simulink model "fusionAlg"  (R2018b)
settings: Solver=FixedStepDiscrete  StartTime=0.0  StopTime=inf  FixedStep=0.01  RelTol=1e-3
PostLoadFcn:
  | if any(exist('dsrtsu_mdlpostloadfcn', 'file') ~= 0), dsrtsu_mdlpostloadfcn('Execute', bdroot); end
model workspace (MAT data in the model file):
  handle : class17 (value not decoded)
(part 5 of 24)

== system fusionAlg/FUSION /FUS_DataAdapter/VisionAdapter/LaneAdapter/Lane_ProtA ==
  EyeQ4_ProtA : Inport
  Bus Creator1 : BusCreator  Inputs=15  OutDataTypeStr=Bus: FUS_EYEQ4_LANE_PROT_ST  NonVirtualBus=on
      settings: InheritFromInputs=off
  Bus Selector : BusSelector  OutputSignals=LH_Line_First_C0,LH_Line_First_C1,LH_Line_First_C2,LH_Line_First_C3,LH_side,LH_First_VR_Start,LH_First_VR_End,LH_Track_ID,LH_Color,LH_Marker_Width,LH_Marker_Width_STD,LH_Existence_Probability,LH_Lanemark_Type,LH_Lanemark_Type_Conf,LH_DLM_Type
  Data Type Conversion{,1..5} (6 alike) : DataTypeConversion  OutDataTypeStr=uint32
  Lane_ProtA_st : Outport  OutDataTypeStr=Bus: FUS_EYEQ4_LANE_PROT_ST
  wires:
  Bus Creator1/1 -> Lane_ProtA_st/1
  Bus Selector/1 -> Bus Creator1/1  "<LH_Line_First_C0>"
  Bus Selector/2 -> Bus Creator1/2  "<LH_Line_First_C1>"
  Bus Selector/3 -> Bus Creator1/3  "<LH_Line_First_C2>"
  Bus Selector/4 -> Bus Creator1/4  "<LH_Line_First_C3>"
  Bus Selector/5 -> Data Type Conversion/1  "<LH_side>"
  Bus Selector/6 -> Bus Creator1/6  "<LH_First_VR_Start>"
  Bus Selector/7 -> Bus Creator1/7  "<LH_First_VR_End>"
  Bus Selector/8 -> Data Type Conversion1/1  "<LH_Track_ID>"
  Bus Selector/9 -> Data Type Conversion2/1  "<LH_Color>"
  Bus Selector/11 -> Bus Creator1/11  "<LH_Marker_Width_STD>"
  Bus Selector/13 -> Data Type Conversion3/1  "<LH_Lanemark_Type>"
  Bus Selector/14 -> Data Type Conversion4/1  "<LH_Lanemark_Type_Conf>"
  Data Type Conversion/1 -> Bus Creator1/5  "LH_Side"
  Data Type Conversion1/1 -> Bus Creator1/8  "LH_Track_ID"
  Data Type Conversion2/1 -> Bus Creator1/9  "LH_Color"
  Data Type Conversion3/1 -> Bus Creator1/13  "LH_Lanemark_Type"
  Data Type Conversion4/1 -> Bus Creator1/14  "LH_Lanemark_Type_Conf"
  EyeQ4_ProtA/1 -> Bus Selector/1
  Bus Selector/15 -> Data Type Conversion5/1  "<LH_DLM_Type>"
  Data Type Conversion5/1 -> Bus Creator1/15  "LH_DLM_Type"
  Bus Selector/12 -> Bus Creator1/12  "<LH_Existence_Probability>"
  Bus Selector/10 -> Bus Creator1/10  "<LH_Marker_Width>"

== system fusionAlg/FUSION /FUS_DataAdapter/VisionAdapter/LaneAdapter/Lane_ProtB ==
  EyeQ4_ProtB : Inport
  Bus Creator1 : BusCreator  Inputs=15  OutDataTypeStr=Bus: FUS_EYEQ4_LANE_PROT_ST  NonVirtualBus=on
      settings: InheritFromInputs=off
  Bus Selector : BusSelector  OutputSignals=LH_Line_First_C0,LH_Line_First_C1,LH_Line_First_C2,LH_Line_First_C3,LH_side,LH_First_VR_Start,LH_First_VR_End,LH_Track_ID,LH_Color,LH_Marker_Width,LH_Marker_Width_STD,LH_Existence_Probability,LH_Lanemark_Type,LH_Lanemark_Type_Conf,LH_DLM_Type
  Data Type Conversion{,1..5} (6 alike) : DataTypeConversion  OutDataTypeStr=uint32
  Lane_ProtB_st : Outport  OutDataTypeStr=Bus: FUS_EYEQ4_LANE_PROT_ST
  wires:
  Bus Creator1/1 -> Lane_ProtB_st/1
  EyeQ4_ProtB/1 -> Bus Selector/1
  Bus Selector/1 -> Bus Creator1/1  "<LH_Line_First_C0>"
  Bus Selector/2 -> Bus Creator1/2  "<LH_Line_First_C1>"
  Bus Selector/3 -> Bus Creator1/3  "<LH_Line_First_C2>"
  Bus Selector/4 -> Bus Creator1/4  "<LH_Line_First_C3>"
  Bus Selector/5 -> Data Type Conversion/1  "<LH_side>"
  Bus Selector/6 -> Bus Creator1/6  "<LH_First_VR_Start>"
  Bus Selector/7 -> Bus Creator1/7  "<LH_First_VR_End>"
  Bus Selector/8 -> Data Type Conversion1/1  "<LH_Track_ID>"
  Bus Selector/9 -> Data Type Conversion2/1  "<LH_Color>"
  Bus Selector/10 -> Bus Creator1/10  "<LH_Marker_Width>"
  Bus Selector/11 -> Bus Creator1/11  "<LH_Marker_Width_STD>"
  Bus Selector/12 -> Bus Creator1/12  "<LH_Existence_Probability>"
  Bus Selector/13 -> Data Type Conversion3/1  "<LH_Lanemark_Type>"
  Bus Selector/14 -> Data Type Conversion4/1  "<LH_Lanemark_Type_Conf>"
  Data Type Conversion/1 -> Bus Creator1/5  "LH_Side"
  Data Type Conversion1/1 -> Bus Creator1/8  "LH_Track_ID"
  Data Type Conversion2/1 -> Bus Creator1/9  "LH_Color"
  Data Type Conversion3/1 -> Bus Creator1/13  "LH_Lanemark_Type"
  Data Type Conversion4/1 -> Bus Creator1/14  "LH_Lanemark_Type_Conf"
  Bus Selector/15 -> Data Type Conversion5/1  "<LH_DLM_Type>"
  Data Type Conversion5/1 -> Bus Creator1/15  "LH_DLM_Type"

== system fusionAlg/FUSION /FUS_DataAdapter/VisionAdapter/LaneAdapter/Lane_Prot_Header ==
  <Host_Prot_Header> : Inport
  Bus Creator1 : BusCreator  Inputs=4  OutDataTypeStr=Bus: FUS_EYEQ4_LANE_PROT_HEADER_ST  NonVirtualBus=on
      settings: InheritFromInputs=off
  Bus Selector : BusSelector  OutputSignals=LH_Sync_ID,LH_Lanes_Count,LH_Estimated_Width,LH_Sonw_On_Road_Prob
  Data Type Conversion : DataTypeConversion  OutDataTypeStr=uint32
  Data Type Conversion1 : DataTypeConversion  OutDataTypeStr=uint32
  HostProtHeader : Outport
  wires:
  Bus Creator1/1 -> HostProtHeader/1
  <Host_Prot_Header>/1 -> Bus Selector/1
  Bus Selector/1 -> Data Type Conversion/1  "<LH_Sync_ID>"
  Bus Selector/2 -> Data Type Conversion1/1  "<LH_Lanes_Count>"
  Bus Selector/3 -> Bus Creator1/3  "<LH_Estimated_Width>"
  Bus Selector/4 -> Bus Creator1/4  "<LH_Sonw_On_Road_Prob>"
  Data Type Conversion/1 -> Bus Creator1/1  "SyncID"
  Data Type Conversion1/1 -> Bus Creator1/2  "LaneCount"

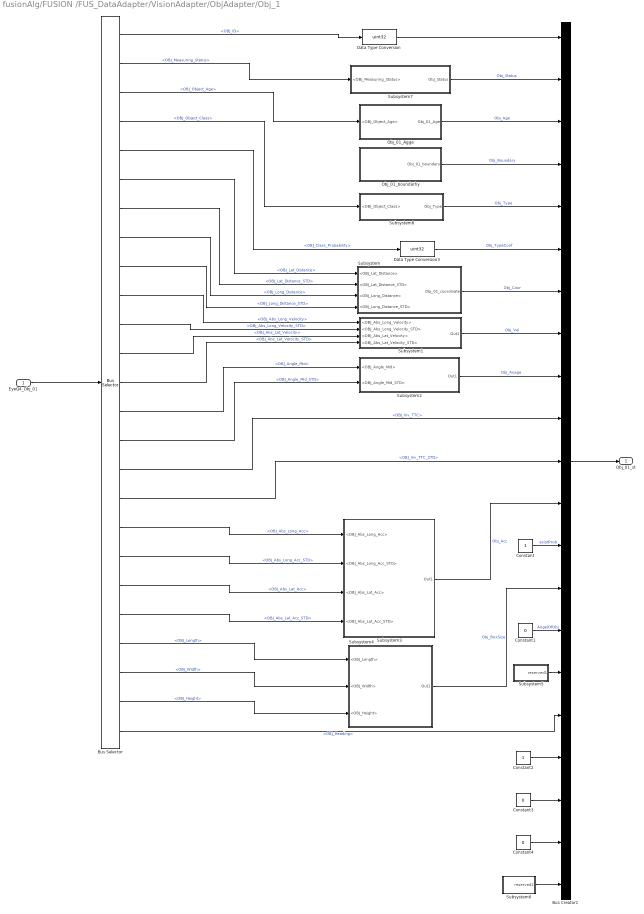
== system fusionAlg/FUSION /FUS_DataAdapter/VisionAdapter/ObjAdapter/Obj_1 ==
  EyeQ4_Obj_01 : Inport
  Bus Creator1 : BusCreator  Inputs=21  OutDataTypeStr=Bus: FUS_VISION_OBJ_ST
      settings: InheritFromInputs=off
  Bus Selector : BusSelector  OutputSignals=OBJ_ID,OBJ_Measuring_Status,OBJ_Object_Age,OBJ_Object_Class,OBJ_Class_Probability,OBJ_Lat_Distance,OBJ_Lat_Distance_STD,OBJ_Long_Distance,OBJ_Long_Distance_STD,OBJ_Abs_Long_Velocity,OBJ_Abs_Long_Velocity_STD,OBJ_Abs_Lat_Velocity,OBJ_Abs_Lat_Velocity_STD,OBJ_Angle_Mid,OBJ_Angle_Mid_STD,OBJ_Inv_TTC,OBJ_Inv_TTC_STD,OBJ_Abs_Long_Acc,OBJ_Abs_Long_Acc_STD,OBJ_Abs_Lat_Acc,OBJ_Abs_Lat_Acc_STD,OBJ_Length,OBJ_Width,OBJ_Height,OBJ_Heading
  Constant : Constant  OutDataTypeStr=single
  Constant1 : Constant  Value=0  OutDataTypeStr=uint8
  Constant2 : Constant  OutDataTypeStr=single
  Constant3 : Constant  Value=0  OutDataTypeStr=single
  Constant4 : Constant  Value=0  OutDataTypeStr=single
  Data Type Conversion : DataTypeConversion  OutDataTypeStr=uint32
  Data Type Conversion3 : DataTypeConversion  OutDataTypeStr=uint32
  Obj_01_Agge : Subsystem
  Obj_01_boundarhy : Subsystem
  Subsystem : Subsystem
  Subsystem1 : Subsystem
  Subsystem2 : Subsystem
  Subsystem3 : Subsystem
  Subsystem4 : Subsystem
  Subsystem5 : Subsystem
  Subsystem6 : Subsystem
  Subsystem7 : Subsystem
  Subsystem8 : Subsystem
  Obj_01_st : Outport  OutDataTypeStr=Bus: FUS_VISION_OBJ_ST
  wires:
  Bus Selector/1 -> Data Type Conversion/1  "<OBJ_ID>"
  Bus Selector/3 -> Obj_01_Agge/1(<OBJ_Object_Age>)  "<OBJ_Object_Age>"
  Obj_01_Agge/1(Obj_01_Age) -> Bus Creator1/3  "Obj_Age"
  Obj_01_boundarhy/1(Obj_01_boundary) -> Bus Creator1/4  "Obj_Boundary"
  Bus Selector/5 -> Data Type Conversion3/1  "<OBJ_Class_Probability>"
  Bus Selector/6 -> Subsystem/1(<OBJ_Lat_Distance>)  "<OBJ_Lat_Distance>"
  Bus Selector/7 -> Subsystem/2(<OBJ_Lat_Distance_STD>)  "<OBJ_Lat_Distance_STD>"
  Bus Selector/8 -> Subsystem/3(<OBJ_Long_Distance>)  "<OBJ_Long_Distance>"
  Bus Selector/9 -> Subsystem/4(<OBJ_Long_Distance_STD>)  "<OBJ_Long_Distance_STD>"
  Subsystem/1(Obj_01_coordinate) -> Bus Creator1/7  "Obj_Coor"
  Bus Selector/10 -> Subsystem1/1(<OBJ_Abs_Long_Velocity>)  "<OBJ_Abs_Long_Velocity>"
  Bus Selector/11 -> Subsystem1/2(<OBJ_Abs_Long_Velocity_STD>)  "<OBJ_Abs_Long_Velocity_STD>"
  Bus Selector/12 -> Subsystem1/3(<OBJ_Abs_Lat_Velocity>)  "<OBJ_Abs_Lat_Velocity>"
  Bus Selector/13 -> Subsystem1/4(<OBJ_Abs_Lat_Velocity_STD>)  "<OBJ_Abs_Lat_Velocity_STD>"
  Subsystem1/1(Out1) -> Bus Creator1/8  "Obj_Vel"
  Bus Selector/14 -> Subsystem2/1(<OBJ_Angle_Mid>)  "<OBJ_Angle_Mid>"
  Bus Selector/15 -> Subsystem2/2(<OBJ_Angle_Mid_STD>)  "<OBJ_Angle_Mid_STD>"
  Subsystem2/1(Out1) -> Bus Creator1/9  "Obj_Anage"
  Bus Selector/16 -> Bus Creator1/10  "<OBJ_Inv_TTC>"
  Bus Selector/17 -> Bus Creator1/11  "<OBJ_Inv_TTC_STD>"
  Bus Selector/18 -> Subsystem3/1(<OBJ_Abs_Long_Acc>)  "<OBJ_Abs_Long_Acc>"
  Bus Selector/19 -> Subsystem3/2(<OBJ_Abs_Long_Acc_STD>)  "<OBJ_Abs_Long_Acc_STD>"
  Bus Selector/20 -> Subsystem3/3(<OBJ_Abs_Lat_Acc>)  "<OBJ_Abs_Lat_Acc>"
  Bus Selector/21 -> Subsystem3/4(<OBJ_Abs_Lat_Acc_STD>)  "<OBJ_Abs_Lat_Acc_STD>"
  Subsystem3/1(Out1) -> Bus Creator1/12  "Obj_Acc"
  Constant/1 -> Bus Creator1/13  "existProb"
  Bus Selector/22 -> Subsystem4/1(<OBJ_Length>)  "<OBJ_Length>"
  Bus Selector/23 -> Subsystem4/2(<OBJ_Width>)  "<OBJ_Width>"
  Bus Selector/24 -> Subsystem4/3(<OBJ_Height>)  "<OBJ_Height>"
  Subsystem4/1(Out1) -> Bus Creator1/14  "Obj_BoxSize"
  Constant1/1 -> Bus Creator1/15  "AngelOfObj"
  Subsystem5/1(reserved1) -> Bus Creator1/16
  Bus Selector/25 -> Bus Creator1/17  "<OBJ_Heading>"
  Constant2/1 -> Bus Creator1/18
  Constant3/1 -> Bus Creator1/19
  Constant4/1 -> Bus Creator1/20
  Subsystem6/1(reserved2) -> Bus Creator1/21
  EyeQ4_Obj_01/1 -> Bus Selector/1
  Bus Creator1/1 -> Obj_01_st/1
  Data Type Conversion/1 -> Bus Creator1/1
  Data Type Conversion3/1 -> Bus Creator1/6  "Obj_TypeConf"
  Bus Selector/2 -> Subsystem7/1(<OBJ_Measuring_Status>)  "<OBJ_Measuring_Status>"
  Subsystem7/1(Obj_Status) -> Bus Creator1/2  "Obj_Status"
  Bus Selector/4 -> Subsystem8/1(<OBJ_Object_Class>)  "<OBJ_Object_Class>"
  Subsystem8/1(Obj_Type) -> Bus Creator1/5  "Obj_Type"

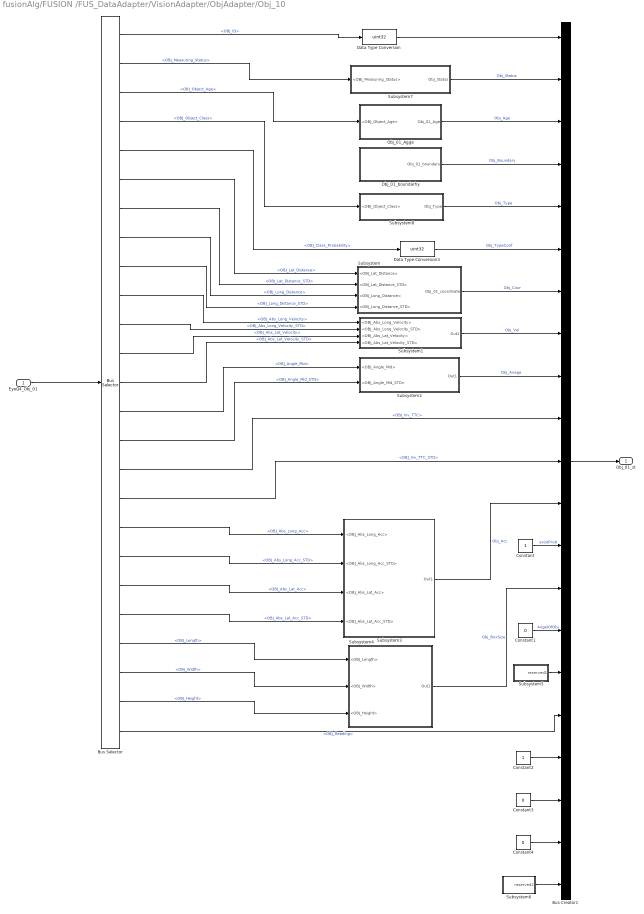
== system fusionAlg/FUSION /FUS_DataAdapter/VisionAdapter/ObjAdapter/Obj_10 ==
  EyeQ4_Obj_01 : Inport
  Bus Creator1 : BusCreator  Inputs=21  OutDataTypeStr=Bus: FUS_VISION_OBJ_ST
      settings: InheritFromInputs=off
  Bus Selector : BusSelector  OutputSignals=OBJ_ID,OBJ_Measuring_Status,OBJ_Object_Age,OBJ_Object_Class,OBJ_Class_Probability,OBJ_Lat_Distance,OBJ_Lat_Distance_STD,OBJ_Long_Distance,OBJ_Long_Distance_STD,OBJ_Abs_Long_Velocity,OBJ_Abs_Long_Velocity_STD,OBJ_Abs_Lat_Velocity,OBJ_Abs_Lat_Velocity_STD,OBJ_Angle_Mid,OBJ_Angle_Mid_STD,OBJ_Inv_TTC,OBJ_Inv_TTC_STD,OBJ_Abs_Long_Acc,OBJ_Abs_Long_Acc_STD,OBJ_Abs_Lat_Acc,OBJ_Abs_Lat_Acc_STD,OBJ_Length,OBJ_Width,OBJ_Height,OBJ_Heading
  Constant : Constant  OutDataTypeStr=single
  Constant1 : Constant  Value=0  OutDataTypeStr=uint8
  Constant2 : Constant  OutDataTypeStr=single
  Constant3 : Constant  Value=0  OutDataTypeStr=single
  Constant4 : Constant  Value=0  OutDataTypeStr=single
  Data Type Conversion : DataTypeConversion  OutDataTypeStr=uint32
  Data Type Conversion3 : DataTypeConversion  OutDataTypeStr=uint32
  Obj_01_Agge : Subsystem
  Obj_01_boundarhy : Subsystem
  Subsystem : Subsystem
  Subsystem1 : Subsystem
  Subsystem2 : Subsystem
  Subsystem3 : Subsystem
  Subsystem4 : Subsystem
  Subsystem5 : Subsystem
  Subsystem6 : Subsystem
  Subsystem7 : Subsystem
  Subsystem8 : Subsystem
  Obj_01_st : Outport  OutDataTypeStr=Bus: FUS_VISION_OBJ_ST
  wires:
  Bus Selector/1 -> Data Type Conversion/1  "<OBJ_ID>"
  Bus Selector/3 -> Obj_01_Agge/1(<OBJ_Object_Age>)  "<OBJ_Object_Age>"
  Obj_01_Agge/1(Obj_01_Age) -> Bus Creator1/3  "Obj_Age"
  Obj_01_boundarhy/1(Obj_01_boundary) -> Bus Creator1/4  "Obj_Boundary"
  Bus Selector/5 -> Data Type Conversion3/1  "<OBJ_Class_Probability>"
  Bus Selector/6 -> Subsystem/1(<OBJ_Lat_Distance>)  "<OBJ_Lat_Distance>"
  Bus Selector/7 -> Subsystem/2(<OBJ_Lat_Distance_STD>)  "<OBJ_Lat_Distance_STD>"
  Bus Selector/8 -> Subsystem/3(<OBJ_Long_Distance>)  "<OBJ_Long_Distance>"
  Bus Selector/9 -> Subsystem/4(<OBJ_Long_Distance_STD>)  "<OBJ_Long_Distance_STD>"
  Subsystem/1(Obj_01_coordinate) -> Bus Creator1/7  "Obj_Coor"
  Bus Selector/10 -> Subsystem1/1(<OBJ_Abs_Long_Velocity>)  "<OBJ_Abs_Long_Velocity>"
  Bus Selector/11 -> Subsystem1/2(<OBJ_Abs_Long_Velocity_STD>)  "<OBJ_Abs_Long_Velocity_STD>"
  Bus Selector/12 -> Subsystem1/3(<OBJ_Abs_Lat_Velocity>)  "<OBJ_Abs_Lat_Velocity>"
  Bus Selector/13 -> Subsystem1/4(<OBJ_Abs_Lat_Velocity_STD>)  "<OBJ_Abs_Lat_Velocity_STD>"
  Subsystem1/1(Out1) -> Bus Creator1/8  "Obj_Vel"
  Bus Selector/14 -> Subsystem2/1(<OBJ_Angle_Mid>)  "<OBJ_Angle_Mid>"
  Bus Selector/15 -> Subsystem2/2(<OBJ_Angle_Mid_STD>)  "<OBJ_Angle_Mid_STD>"
  Subsystem2/1(Out1) -> Bus Creator1/9  "Obj_Anage"
  Bus Selector/16 -> Bus Creator1/10  "<OBJ_Inv_TTC>"
  Bus Selector/17 -> Bus Creator1/11  "<OBJ_Inv_TTC_STD>"
  Bus Selector/18 -> Subsystem3/1(<OBJ_Abs_Long_Acc>)  "<OBJ_Abs_Long_Acc>"
  Bus Selector/19 -> Subsystem3/2(<OBJ_Abs_Long_Acc_STD>)  "<OBJ_Abs_Long_Acc_STD>"
  Bus Selector/20 -> Subsystem3/3(<OBJ_Abs_Lat_Acc>)  "<OBJ_Abs_Lat_Acc>"
  Bus Selector/21 -> Subsystem3/4(<OBJ_Abs_Lat_Acc_STD>)  "<OBJ_Abs_Lat_Acc_STD>"
  Subsystem3/1(Out1) -> Bus Creator1/12  "Obj_Acc"
  Constant/1 -> Bus Creator1/13  "existProb"
  Bus Selector/22 -> Subsystem4/1(<OBJ_Length>)  "<OBJ_Length>"
  Bus Selector/23 -> Subsystem4/2(<OBJ_Width>)  "<OBJ_Width>"
  Bus Selector/24 -> Subsystem4/3(<OBJ_Height>)  "<OBJ_Height>"
  Subsystem4/1(Out1) -> Bus Creator1/14  "Obj_BoxSize"
  Constant1/1 -> Bus Creator1/15  "AngelOfObj"
  Subsystem5/1(reserved1) -> Bus Creator1/16
  Bus Selector/25 -> Bus Creator1/17  "<OBJ_Heading>"
  Constant2/1 -> Bus Creator1/18
  Constant3/1 -> Bus Creator1/19
  Constant4/1 -> Bus Creator1/20
  Subsystem6/1(reserved2) -> Bus Creator1/21
  EyeQ4_Obj_01/1 -> Bus Selector/1
  Bus Creator1/1 -> Obj_01_st/1
  Data Type Conversion/1 -> Bus Creator1/1
  Data Type Conversion3/1 -> Bus Creator1/6  "Obj_TypeConf"
  Bus Selector/2 -> Subsystem7/1(<OBJ_Measuring_Status>)  "<OBJ_Measuring_Status>"
  Subsystem7/1(Obj_Status) -> Bus Creator1/2  "Obj_Status"
  Bus Selector/4 -> Subsystem8/1(<OBJ_Object_Class>)  "<OBJ_Object_Class>"
  Subsystem8/1(Obj_Type) -> Bus Creator1/5  "Obj_Type"

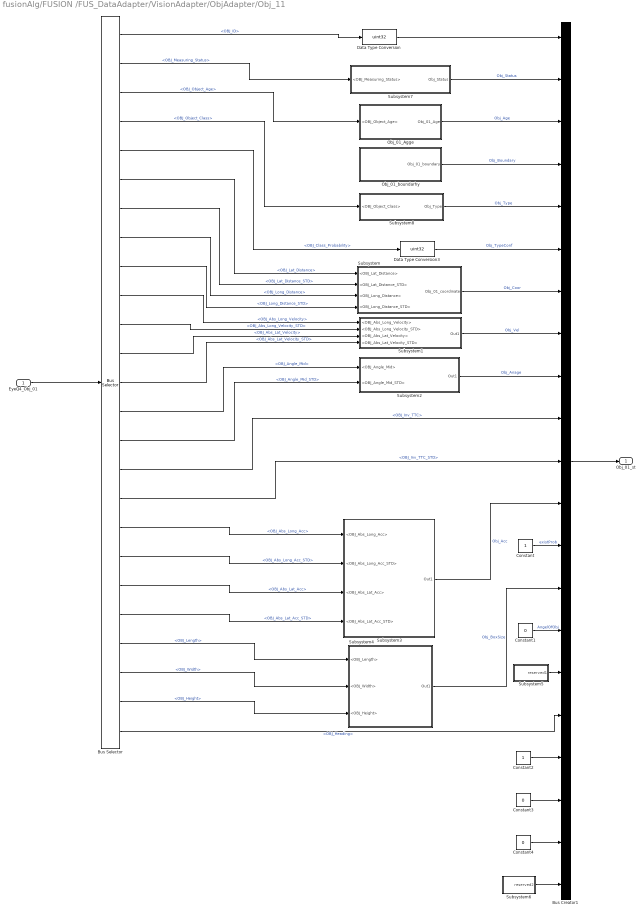
== system fusionAlg/FUSION /FUS_DataAdapter/VisionAdapter/ObjAdapter/Obj_11 ==
  EyeQ4_Obj_01 : Inport
  Bus Creator1 : BusCreator  Inputs=21  OutDataTypeStr=Bus: FUS_VISION_OBJ_ST
      settings: InheritFromInputs=off
  Bus Selector : BusSelector  OutputSignals=OBJ_ID,OBJ_Measuring_Status,OBJ_Object_Age,OBJ_Object_Class,OBJ_Class_Probability,OBJ_Lat_Distance,OBJ_Lat_Distance_STD,OBJ_Long_Distance,OBJ_Long_Distance_STD,OBJ_Abs_Long_Velocity,OBJ_Abs_Long_Velocity_STD,OBJ_Abs_Lat_Velocity,OBJ_Abs_Lat_Velocity_STD,OBJ_Angle_Mid,OBJ_Angle_Mid_STD,OBJ_Inv_TTC,OBJ_Inv_TTC_STD,OBJ_Abs_Long_Acc,OBJ_Abs_Long_Acc_STD,OBJ_Abs_Lat_Acc,OBJ_Abs_Lat_Acc_STD,OBJ_Length,OBJ_Width,OBJ_Height,OBJ_Heading
  Constant : Constant  OutDataTypeStr=single
  Constant1 : Constant  Value=0  OutDataTypeStr=uint8
  Constant2 : Constant  OutDataTypeStr=single
  Constant3 : Constant  Value=0  OutDataTypeStr=single
  Constant4 : Constant  Value=0  OutDataTypeStr=single
  Data Type Conversion : DataTypeConversion  OutDataTypeStr=uint32
  Data Type Conversion3 : DataTypeConversion  OutDataTypeStr=uint32
  Obj_01_Agge : Subsystem
  Obj_01_boundarhy : Subsystem
  Subsystem : Subsystem
  Subsystem1 : Subsystem
  Subsystem2 : Subsystem
  Subsystem3 : Subsystem
  Subsystem4 : Subsystem
  Subsystem5 : Subsystem
  Subsystem6 : Subsystem
  Subsystem7 : Subsystem
  Subsystem8 : Subsystem
  Obj_01_st : Outport  OutDataTypeStr=Bus: FUS_VISION_OBJ_ST
  wires:
  Bus Selector/1 -> Data Type Conversion/1  "<OBJ_ID>"
  Bus Selector/3 -> Obj_01_Agge/1(<OBJ_Object_Age>)  "<OBJ_Object_Age>"
  Obj_01_Agge/1(Obj_01_Age) -> Bus Creator1/3  "Obj_Age"
  Obj_01_boundarhy/1(Obj_01_boundary) -> Bus Creator1/4  "Obj_Boundary"
  Bus Selector/5 -> Data Type Conversion3/1  "<OBJ_Class_Probability>"
  Bus Selector/6 -> Subsystem/1(<OBJ_Lat_Distance>)  "<OBJ_Lat_Distance>"
  Bus Selector/7 -> Subsystem/2(<OBJ_Lat_Distance_STD>)  "<OBJ_Lat_Distance_STD>"
  Bus Selector/8 -> Subsystem/3(<OBJ_Long_Distance>)  "<OBJ_Long_Distance>"
  Bus Selector/9 -> Subsystem/4(<OBJ_Long_Distance_STD>)  "<OBJ_Long_Distance_STD>"
  Subsystem/1(Obj_01_coordinate) -> Bus Creator1/7  "Obj_Coor"
  Bus Selector/10 -> Subsystem1/1(<OBJ_Abs_Long_Velocity>)  "<OBJ_Abs_Long_Velocity>"
  Bus Selector/11 -> Subsystem1/2(<OBJ_Abs_Long_Velocity_STD>)  "<OBJ_Abs_Long_Velocity_STD>"
  Bus Selector/12 -> Subsystem1/3(<OBJ_Abs_Lat_Velocity>)  "<OBJ_Abs_Lat_Velocity>"
  Bus Selector/13 -> Subsystem1/4(<OBJ_Abs_Lat_Velocity_STD>)  "<OBJ_Abs_Lat_Velocity_STD>"
  Subsystem1/1(Out1) -> Bus Creator1/8  "Obj_Vel"
  Bus Selector/14 -> Subsystem2/1(<OBJ_Angle_Mid>)  "<OBJ_Angle_Mid>"
  Bus Selector/15 -> Subsystem2/2(<OBJ_Angle_Mid_STD>)  "<OBJ_Angle_Mid_STD>"
  Subsystem2/1(Out1) -> Bus Creator1/9  "Obj_Anage"
  Bus Selector/16 -> Bus Creator1/10  "<OBJ_Inv_TTC>"
  Bus Selector/17 -> Bus Creator1/11  "<OBJ_Inv_TTC_STD>"
  Bus Selector/18 -> Subsystem3/1(<OBJ_Abs_Long_Acc>)  "<OBJ_Abs_Long_Acc>"
  Bus Selector/19 -> Subsystem3/2(<OBJ_Abs_Long_Acc_STD>)  "<OBJ_Abs_Long_Acc_STD>"
  Bus Selector/20 -> Subsystem3/3(<OBJ_Abs_Lat_Acc>)  "<OBJ_Abs_Lat_Acc>"
  Bus Selector/21 -> Subsystem3/4(<OBJ_Abs_Lat_Acc_STD>)  "<OBJ_Abs_Lat_Acc_STD>"
  Subsystem3/1(Out1) -> Bus Creator1/12  "Obj_Acc"
  Constant/1 -> Bus Creator1/13  "existProb"
  Bus Selector/22 -> Subsystem4/1(<OBJ_Length>)  "<OBJ_Length>"
  Bus Selector/23 -> Subsystem4/2(<OBJ_Width>)  "<OBJ_Width>"
  Bus Selector/24 -> Subsystem4/3(<OBJ_Height>)  "<OBJ_Height>"
  Subsystem4/1(Out1) -> Bus Creator1/14  "Obj_BoxSize"
  Constant1/1 -> Bus Creator1/15  "AngelOfObj"
  Subsystem5/1(reserved1) -> Bus Creator1/16
  Bus Selector/25 -> Bus Creator1/17  "<OBJ_Heading>"
  Constant2/1 -> Bus Creator1/18
  Constant3/1 -> Bus Creator1/19
  Constant4/1 -> Bus Creator1/20
  Subsystem6/1(reserved2) -> Bus Creator1/21
  EyeQ4_Obj_01/1 -> Bus Selector/1
  Bus Creator1/1 -> Obj_01_st/1
  Data Type Conversion/1 -> Bus Creator1/1
  Data Type Conversion3/1 -> Bus Creator1/6  "Obj_TypeConf"
  Bus Selector/2 -> Subsystem7/1(<OBJ_Measuring_Status>)  "<OBJ_Measuring_Status>"
  Subsystem7/1(Obj_Status) -> Bus Creator1/2  "Obj_Status"
  Bus Selector/4 -> Subsystem8/1(<OBJ_Object_Class>)  "<OBJ_Object_Class>"
  Subsystem8/1(Obj_Type) -> Bus Creator1/5  "Obj_Type"

== system fusionAlg/FUSION /FUS_DataAdapter/VisionAdapter/ObjAdapter/Obj_12 ==
  EyeQ4_Obj_01 : Inport
  Bus Creator1 : BusCreator  Inputs=21  OutDataTypeStr=Bus: FUS_VISION_OBJ_ST
      settings: InheritFromInputs=off
  Bus Selector : BusSelector  OutputSignals=OBJ_ID,OBJ_Measuring_Status,OBJ_Object_Age,OBJ_Object_Class,OBJ_Class_Probability,OBJ_Lat_Distance,OBJ_Lat_Distance_STD,OBJ_Long_Distance,OBJ_Long_Distance_STD,OBJ_Abs_Long_Velocity,OBJ_Abs_Long_Velocity_STD,OBJ_Abs_Lat_Velocity,OBJ_Abs_Lat_Velocity_STD,OBJ_Angle_Mid,OBJ_Angle_Mid_STD,OBJ_Inv_TTC,OBJ_Inv_TTC_STD,OBJ_Abs_Long_Acc,OBJ_Abs_Long_Acc_STD,OBJ_Abs_Lat_Acc,OBJ_Abs_Lat_Acc_STD,OBJ_Length,OBJ_Width,OBJ_Height,OBJ_Heading
  Constant : Constant  OutDataTypeStr=single
  Constant1 : Constant  Value=0  OutDataTypeStr=uint8
  Constant2 : Constant  OutDataTypeStr=single
  Constant3 : Constant  Value=0  OutDataTypeStr=single
  Constant4 : Constant  Value=0  OutDataTypeStr=single
  Data Type Conversion : DataTypeConversion  OutDataTypeStr=uint32
  Data Type Conversion3 : DataTypeConversion  OutDataTypeStr=uint32
  Obj_01_Agge : Subsystem
  Obj_01_boundarhy : Subsystem
  Subsystem : Subsystem
  Subsystem1 : Subsystem
  Subsystem2 : Subsystem
  Subsystem3 : Subsystem
  Subsystem4 : Subsystem
  Subsystem5 : Subsystem
  Subsystem6 : Subsystem
  Subsystem7 : Subsystem
  Subsystem8 : Subsystem
  Obj_01_st : Outport  OutDataTypeStr=Bus: FUS_VISION_OBJ_ST
  wires:
  Bus Selector/1 -> Data Type Conversion/1  "<OBJ_ID>"
  Bus Selector/3 -> Obj_01_Agge/1(<OBJ_Object_Age>)  "<OBJ_Object_Age>"
  Obj_01_Agge/1(Obj_01_Age) -> Bus Creator1/3  "Obj_Age"
  Obj_01_boundarhy/1(Obj_01_boundary) -> Bus Creator1/4  "Obj_Boundary"
  Bus Selector/5 -> Data Type Conversion3/1  "<OBJ_Class_Probability>"
  Bus Selector/6 -> Subsystem/1(<OBJ_Lat_Distance>)  "<OBJ_Lat_Distance>"
  Bus Selector/7 -> Subsystem/2(<OBJ_Lat_Distance_STD>)  "<OBJ_Lat_Distance_STD>"
  Bus Selector/8 -> Subsystem/3(<OBJ_Long_Distance>)  "<OBJ_Long_Distance>"
  Bus Selector/9 -> Subsystem/4(<OBJ_Long_Distance_STD>)  "<OBJ_Long_Distance_STD>"
  Subsystem/1(Obj_01_coordinate) -> Bus Creator1/7  "Obj_Coor"
  Bus Selector/10 -> Subsystem1/1(<OBJ_Abs_Long_Velocity>)  "<OBJ_Abs_Long_Velocity>"
  Bus Selector/11 -> Subsystem1/2(<OBJ_Abs_Long_Velocity_STD>)  "<OBJ_Abs_Long_Velocity_STD>"
  Bus Selector/12 -> Subsystem1/3(<OBJ_Abs_Lat_Velocity>)  "<OBJ_Abs_Lat_Velocity>"
  Bus Selector/13 -> Subsystem1/4(<OBJ_Abs_Lat_Velocity_STD>)  "<OBJ_Abs_Lat_Velocity_STD>"
  Subsystem1/1(Out1) -> Bus Creator1/8  "Obj_Vel"
  Bus Selector/14 -> Subsystem2/1(<OBJ_Angle_Mid>)  "<OBJ_Angle_Mid>"
  Bus Selector/15 -> Subsystem2/2(<OBJ_Angle_Mid_STD>)  "<OBJ_Angle_Mid_STD>"
  Subsystem2/1(Out1) -> Bus Creator1/9  "Obj_Anage"
  Bus Selector/16 -> Bus Creator1/10  "<OBJ_Inv_TTC>"
  Bus Selector/17 -> Bus Creator1/11  "<OBJ_Inv_TTC_STD>"
  Bus Selector/18 -> Subsystem3/1(<OBJ_Abs_Long_Acc>)  "<OBJ_Abs_Long_Acc>"
  Bus Selector/19 -> Subsystem3/2(<OBJ_Abs_Long_Acc_STD>)  "<OBJ_Abs_Long_Acc_STD>"
  Bus Selector/20 -> Subsystem3/3(<OBJ_Abs_Lat_Acc>)  "<OBJ_Abs_Lat_Acc>"
  Bus Selector/21 -> Subsystem3/4(<OBJ_Abs_Lat_Acc_STD>)  "<OBJ_Abs_Lat_Acc_STD>"
  Subsystem3/1(Out1) -> Bus Creator1/12  "Obj_Acc"
  Constant/1 -> Bus Creator1/13  "existProb"
  Bus Selector/22 -> Subsystem4/1(<OBJ_Length>)  "<OBJ_Length>"
  Bus Selector/23 -> Subsystem4/2(<OBJ_Width>)  "<OBJ_Width>"
  Bus Selector/24 -> Subsystem4/3(<OBJ_Height>)  "<OBJ_Height>"
  Subsystem4/1(Out1) -> Bus Creator1/14  "Obj_BoxSize"
  Constant1/1 -> Bus Creator1/15  "AngelOfObj"
  Subsystem5/1(reserved1) -> Bus Creator1/16
  Bus Selector/25 -> Bus Creator1/17  "<OBJ_Heading>"
  Constant2/1 -> Bus Creator1/18
  Constant3/1 -> Bus Creator1/19
  Constant4/1 -> Bus Creator1/20
  Subsystem6/1(reserved2) -> Bus Creator1/21
  EyeQ4_Obj_01/1 -> Bus Selector/1
  Bus Creator1/1 -> Obj_01_st/1
  Data Type Conversion/1 -> Bus Creator1/1
  Data Type Conversion3/1 -> Bus Creator1/6  "Obj_TypeConf"
  Bus Selector/2 -> Subsystem7/1(<OBJ_Measuring_Status>)  "<OBJ_Measuring_Status>"
  Subsystem7/1(Obj_Status) -> Bus Creator1/2  "Obj_Status"
  Bus Selector/4 -> Subsystem8/1(<OBJ_Object_Class>)  "<OBJ_Object_Class>"
  Subsystem8/1(Obj_Type) -> Bus Creator1/5  "Obj_Type"

== system fusionAlg/FUSION /FUS_DataAdapter/VisionAdapter/ObjAdapter/Obj_13 ==
  EyeQ4_Obj_01 : Inport
  Bus Creator1 : BusCreator  Inputs=21  OutDataTypeStr=Bus: FUS_VISION_OBJ_ST
      settings: InheritFromInputs=off
  Bus Selector : BusSelector  OutputSignals=OBJ_ID,OBJ_Measuring_Status,OBJ_Object_Age,OBJ_Object_Class,OBJ_Class_Probability,OBJ_Lat_Distance,OBJ_Lat_Distance_STD,OBJ_Long_Distance,OBJ_Long_Distance_STD,OBJ_Abs_Long_Velocity,OBJ_Abs_Long_Velocity_STD,OBJ_Abs_Lat_Velocity,OBJ_Abs_Lat_Velocity_STD,OBJ_Angle_Mid,OBJ_Angle_Mid_STD,OBJ_Inv_TTC,OBJ_Inv_TTC_STD,OBJ_Abs_Long_Acc,OBJ_Abs_Long_Acc_STD,OBJ_Abs_Lat_Acc,OBJ_Abs_Lat_Acc_STD,OBJ_Length,OBJ_Width,OBJ_Height,OBJ_Heading
  Constant : Constant  OutDataTypeStr=single
  Constant1 : Constant  Value=0  OutDataTypeStr=uint8
  Constant2 : Constant  OutDataTypeStr=single
  Constant3 : Constant  Value=0  OutDataTypeStr=single
  Constant4 : Constant  Value=0  OutDataTypeStr=single
  Data Type Conversion : DataTypeConversion  OutDataTypeStr=uint32
  Data Type Conversion3 : DataTypeConversion  OutDataTypeStr=uint32
  Obj_01_Agge : Subsystem
  Obj_01_boundarhy : Subsystem
  Subsystem : Subsystem
  Subsystem1 : Subsystem
  Subsystem2 : Subsystem
  Subsystem3 : Subsystem
  Subsystem4 : Subsystem
  Subsystem5 : Subsystem
  Subsystem6 : Subsystem
  Subsystem7 : Subsystem
  Subsystem8 : Subsystem
  Obj_01_st : Outport  OutDataTypeStr=Bus: FUS_VISION_OBJ_ST
  wires:
  Bus Selector/1 -> Data Type Conversion/1  "<OBJ_ID>"
  Bus Selector/3 -> Obj_01_Agge/1(<OBJ_Object_Age>)  "<OBJ_Object_Age>"
  Obj_01_Agge/1(Obj_01_Age) -> Bus Creator1/3  "Obj_Age"
  Obj_01_boundarhy/1(Obj_01_boundary) -> Bus Creator1/4  "Obj_Boundary"
  Bus Selector/5 -> Data Type Conversion3/1  "<OBJ_Class_Probability>"
  Bus Selector/6 -> Subsystem/1(<OBJ_Lat_Distance>)  "<OBJ_Lat_Distance>"
  Bus Selector/7 -> Subsystem/2(<OBJ_Lat_Distance_STD>)  "<OBJ_Lat_Distance_STD>"
  Bus Selector/8 -> Subsystem/3(<OBJ_Long_Distance>)  "<OBJ_Long_Distance>"
  Bus Selector/9 -> Subsystem/4(<OBJ_Long_Distance_STD>)  "<OBJ_Long_Distance_STD>"
  Subsystem/1(Obj_01_coordinate) -> Bus Creator1/7  "Obj_Coor"
  Bus Selector/10 -> Subsystem1/1(<OBJ_Abs_Long_Velocity>)  "<OBJ_Abs_Long_Velocity>"
  Bus Selector/11 -> Subsystem1/2(<OBJ_Abs_Long_Velocity_STD>)  "<OBJ_Abs_Long_Velocity_STD>"
  Bus Selector/12 -> Subsystem1/3(<OBJ_Abs_Lat_Velocity>)  "<OBJ_Abs_Lat_Velocity>"
  Bus Selector/13 -> Subsystem1/4(<OBJ_Abs_Lat_Velocity_STD>)  "<OBJ_Abs_Lat_Velocity_STD>"
  Subsystem1/1(Out1) -> Bus Creator1/8  "Obj_Vel"
  Bus Selector/14 -> Subsystem2/1(<OBJ_Angle_Mid>)  "<OBJ_Angle_Mid>"
  Bus Selector/15 -> Subsystem2/2(<OBJ_Angle_Mid_STD>)  "<OBJ_Angle_Mid_STD>"
  Subsystem2/1(Out1) -> Bus Creator1/9  "Obj_Anage"
  Bus Selector/16 -> Bus Creator1/10  "<OBJ_Inv_TTC>"
  Bus Selector/17 -> Bus Creator1/11  "<OBJ_Inv_TTC_STD>"
  Bus Selector/18 -> Subsystem3/1(<OBJ_Abs_Long_Acc>)  "<OBJ_Abs_Long_Acc>"
  Bus Selector/19 -> Subsystem3/2(<OBJ_Abs_Long_Acc_STD>)  "<OBJ_Abs_Long_Acc_STD>"
  Bus Selector/20 -> Subsystem3/3(<OBJ_Abs_Lat_Acc>)  "<OBJ_Abs_Lat_Acc>"
  Bus Selector/21 -> Subsystem3/4(<OBJ_Abs_Lat_Acc_STD>)  "<OBJ_Abs_Lat_Acc_STD>"
  Subsystem3/1(Out1) -> Bus Creator1/12  "Obj_Acc"
  Constant/1 -> Bus Creator1/13  "existProb"
  Bus Selector/22 -> Subsystem4/1(<OBJ_Length>)  "<OBJ_Length>"
  Bus Selector/23 -> Subsystem4/2(<OBJ_Width>)  "<OBJ_Width>"
  Bus Selector/24 -> Subsystem4/3(<OBJ_Height>)  "<OBJ_Height>"
  Subsystem4/1(Out1) -> Bus Creator1/14  "Obj_BoxSize"
  Constant1/1 -> Bus Creator1/15  "AngelOfObj"
  Subsystem5/1(reserved1) -> Bus Creator1/16
  Bus Selector/25 -> Bus Creator1/17  "<OBJ_Heading>"
  Constant2/1 -> Bus Creator1/18
  Constant3/1 -> Bus Creator1/19
  Constant4/1 -> Bus Creator1/20
  Subsystem6/1(reserved2) -> Bus Creator1/21
  EyeQ4_Obj_01/1 -> Bus Selector/1
  Bus Creator1/1 -> Obj_01_st/1
  Data Type Conversion/1 -> Bus Creator1/1
  Data Type Conversion3/1 -> Bus Creator1/6  "Obj_TypeConf"
  Bus Selector/2 -> Subsystem7/1(<OBJ_Measuring_Status>)  "<OBJ_Measuring_Status>"
  Subsystem7/1(Obj_Status) -> Bus Creator1/2  "Obj_Status"
  Bus Selector/4 -> Subsystem8/1(<OBJ_Object_Class>)  "<OBJ_Object_Class>"
  Subsystem8/1(Obj_Type) -> Bus Creator1/5  "Obj_Type"

== system fusionAlg/FUSION /FUS_DataAdapter/VisionAdapter/ObjAdapter/Obj_14 ==
  EyeQ4_Obj_01 : Inport
  Bus Creator1 : BusCreator  Inputs=21  OutDataTypeStr=Bus: FUS_VISION_OBJ_ST
      settings: InheritFromInputs=off
  Bus Selector : BusSelector  OutputSignals=OBJ_ID,OBJ_Measuring_Status,OBJ_Object_Age,OBJ_Object_Class,OBJ_Class_Probability,OBJ_Lat_Distance,OBJ_Lat_Distance_STD,OBJ_Long_Distance,OBJ_Long_Distance_STD,OBJ_Abs_Long_Velocity,OBJ_Abs_Long_Velocity_STD,OBJ_Abs_Lat_Velocity,OBJ_Abs_Lat_Velocity_STD,OBJ_Angle_Mid,OBJ_Angle_Mid_STD,OBJ_Inv_TTC,OBJ_Inv_TTC_STD,OBJ_Abs_Long_Acc,OBJ_Abs_Long_Acc_STD,OBJ_Abs_Lat_Acc,OBJ_Abs_Lat_Acc_STD,OBJ_Length,OBJ_Width,OBJ_Height,OBJ_Heading
  Constant : Constant  OutDataTypeStr=single
  Constant1 : Constant  Value=0  OutDataTypeStr=uint8
  Constant2 : Constant  OutDataTypeStr=single
  Constant3 : Constant  Value=0  OutDataTypeStr=single
  Constant4 : Constant  Value=0  OutDataTypeStr=single
  Data Type Conversion : DataTypeConversion  OutDataTypeStr=uint32
  Data Type Conversion3 : DataTypeConversion  OutDataTypeStr=uint32
  Obj_01_Agge : Subsystem
  Obj_01_boundarhy : Subsystem
  Subsystem : Subsystem
  Subsystem1 : Subsystem
  Subsystem2 : Subsystem
  Subsystem3 : Subsystem
  Subsystem4 : Subsystem
  Subsystem5 : Subsystem
  Subsystem6 : Subsystem
  Subsystem7 : Subsystem
  Subsystem8 : Subsystem
  Obj_01_st : Outport  OutDataTypeStr=Bus: FUS_VISION_OBJ_ST
  wires:
  Bus Selector/1 -> Data Type Conversion/1  "<OBJ_ID>"
  Bus Selector/3 -> Obj_01_Agge/1(<OBJ_Object_Age>)  "<OBJ_Object_Age>"
  Obj_01_Agge/1(Obj_01_Age) -> Bus Creator1/3  "Obj_Age"
  Obj_01_boundarhy/1(Obj_01_boundary) -> Bus Creator1/4  "Obj_Boundary"
  Bus Selector/5 -> Data Type Conversion3/1  "<OBJ_Class_Probability>"
  Bus Selector/6 -> Subsystem/1(<OBJ_Lat_Distance>)  "<OBJ_Lat_Distance>"
  Bus Selector/7 -> Subsystem/2(<OBJ_Lat_Distance_STD>)  "<OBJ_Lat_Distance_STD>"
  Bus Selector/8 -> Subsystem/3(<OBJ_Long_Distance>)  "<OBJ_Long_Distance>"
  Bus Selector/9 -> Subsystem/4(<OBJ_Long_Distance_STD>)  "<OBJ_Long_Distance_STD>"
  Subsystem/1(Obj_01_coordinate) -> Bus Creator1/7  "Obj_Coor"
  Bus Selector/10 -> Subsystem1/1(<OBJ_Abs_Long_Velocity>)  "<OBJ_Abs_Long_Velocity>"
  Bus Selector/11 -> Subsystem1/2(<OBJ_Abs_Long_Velocity_STD>)  "<OBJ_Abs_Long_Velocity_STD>"
  Bus Selector/12 -> Subsystem1/3(<OBJ_Abs_Lat_Velocity>)  "<OBJ_Abs_Lat_Velocity>"
  Bus Selector/13 -> Subsystem1/4(<OBJ_Abs_Lat_Velocity_STD>)  "<OBJ_Abs_Lat_Velocity_STD>"
  Subsystem1/1(Out1) -> Bus Creator1/8  "Obj_Vel"
  Bus Selector/14 -> Subsystem2/1(<OBJ_Angle_Mid>)  "<OBJ_Angle_Mid>"
  Bus Selector/15 -> Subsystem2/2(<OBJ_Angle_Mid_STD>)  "<OBJ_Angle_Mid_STD>"
  Subsystem2/1(Out1) -> Bus Creator1/9  "Obj_Anage"
  Bus Selector/16 -> Bus Creator1/10  "<OBJ_Inv_TTC>"
  Bus Selector/17 -> Bus Creator1/11  "<OBJ_Inv_TTC_STD>"
  Bus Selector/18 -> Subsystem3/1(<OBJ_Abs_Long_Acc>)  "<OBJ_Abs_Long_Acc>"
  Bus Selector/19 -> Subsystem3/2(<OBJ_Abs_Long_Acc_STD>)  "<OBJ_Abs_Long_Acc_STD>"
  Bus Selector/20 -> Subsystem3/3(<OBJ_Abs_Lat_Acc>)  "<OBJ_Abs_Lat_Acc>"
  Bus Selector/21 -> Subsystem3/4(<OBJ_Abs_Lat_Acc_STD>)  "<OBJ_Abs_Lat_Acc_STD>"
  Subsystem3/1(Out1) -> Bus Creator1/12  "Obj_Acc"
  Constant/1 -> Bus Creator1/13  "existProb"
  Bus Selector/22 -> Subsystem4/1(<OBJ_Length>)  "<OBJ_Length>"
  Bus Selector/23 -> Subsystem4/2(<OBJ_Width>)  "<OBJ_Width>"
  Bus Selector/24 -> Subsystem4/3(<OBJ_Height>)  "<OBJ_Height>"
  Subsystem4/1(Out1) -> Bus Creator1/14  "Obj_BoxSize"
  Constant1/1 -> Bus Creator1/15  "AngelOfObj"
  Subsystem5/1(reserved1) -> Bus Creator1/16
  Bus Selector/25 -> Bus Creator1/17  "<OBJ_Heading>"
  Constant2/1 -> Bus Creator1/18
  Constant3/1 -> Bus Creator1/19
  Constant4/1 -> Bus Creator1/20
  Subsystem6/1(reserved2) -> Bus Creator1/21
  EyeQ4_Obj_01/1 -> Bus Selector/1
  Bus Creator1/1 -> Obj_01_st/1
  Data Type Conversion/1 -> Bus Creator1/1
  Data Type Conversion3/1 -> Bus Creator1/6  "Obj_TypeConf"
  Bus Selector/2 -> Subsystem7/1(<OBJ_Measuring_Status>)  "<OBJ_Measuring_Status>"
  Subsystem7/1(Obj_Status) -> Bus Creator1/2  "Obj_Status"
  Bus Selector/4 -> Subsystem8/1(<OBJ_Object_Class>)  "<OBJ_Object_Class>"
  Subsystem8/1(Obj_Type) -> Bus Creator1/5  "Obj_Type"

== system fusionAlg/FUSION /FUS_DataAdapter/VisionAdapter/ObjAdapter/Obj_15 ==
  EyeQ4_Obj_01 : Inport
  Bus Creator1 : BusCreator  Inputs=21  OutDataTypeStr=Bus: FUS_VISION_OBJ_ST
      settings: InheritFromInputs=off
  Bus Selector : BusSelector  OutputSignals=OBJ_ID,OBJ_Measuring_Status,OBJ_Object_Age,OBJ_Object_Class,OBJ_Class_Probability,OBJ_Lat_Distance,OBJ_Lat_Distance_STD,OBJ_Long_Distance,OBJ_Long_Distance_STD,OBJ_Abs_Long_Velocity,OBJ_Abs_Long_Velocity_STD,OBJ_Abs_Lat_Velocity,OBJ_Abs_Lat_Velocity_STD,OBJ_Angle_Mid,OBJ_Angle_Mid_STD,OBJ_Inv_TTC,OBJ_Inv_TTC_STD,OBJ_Abs_Long_Acc,OBJ_Abs_Long_Acc_STD,OBJ_Abs_Lat_Acc,OBJ_Abs_Lat_Acc_STD,OBJ_Length,OBJ_Width,OBJ_Height,OBJ_Heading
  Constant : Constant  OutDataTypeStr=single
  Constant1 : Constant  Value=0  OutDataTypeStr=uint8
  Constant2 : Constant  OutDataTypeStr=single
  Constant3 : Constant  Value=0  OutDataTypeStr=single
  Constant4 : Constant  Value=0  OutDataTypeStr=single
  Data Type Conversion : DataTypeConversion  OutDataTypeStr=uint32
  Data Type Conversion3 : DataTypeConversion  OutDataTypeStr=uint32
  Obj_01_Agge : Subsystem
  Obj_01_boundarhy : Subsystem
  Subsystem : Subsystem
  Subsystem1 : Subsystem
  Subsystem2 : Subsystem
  Subsystem3 : Subsystem
  Subsystem4 : Subsystem
  Subsystem5 : Subsystem
  Subsystem6 : Subsystem
  Subsystem7 : Subsystem
  Subsystem8 : Subsystem
  Obj_01_st : Outport  OutDataTypeStr=Bus: FUS_VISION_OBJ_ST
  wires:
  Bus Selector/1 -> Data Type Conversion/1  "<OBJ_ID>"
  Bus Selector/3 -> Obj_01_Agge/1(<OBJ_Object_Age>)  "<OBJ_Object_Age>"
  Obj_01_Agge/1(Obj_01_Age) -> Bus Creator1/3  "Obj_Age"
  Obj_01_boundarhy/1(Obj_01_boundary) -> Bus Creator1/4  "Obj_Boundary"
  Bus Selector/5 -> Data Type Conversion3/1  "<OBJ_Class_Probability>"
  Bus Selector/6 -> Subsystem/1(<OBJ_Lat_Distance>)  "<OBJ_Lat_Distance>"
  Bus Selector/7 -> Subsystem/2(<OBJ_Lat_Distance_STD>)  "<OBJ_Lat_Distance_STD>"
  Bus Selector/8 -> Subsystem/3(<OBJ_Long_Distance>)  "<OBJ_Long_Distance>"
  Bus Selector/9 -> Subsystem/4(<OBJ_Long_Distance_STD>)  "<OBJ_Long_Distance_STD>"
  Subsystem/1(Obj_01_coordinate) -> Bus Creator1/7  "Obj_Coor"
  Bus Selector/10 -> Subsystem1/1(<OBJ_Abs_Long_Velocity>)  "<OBJ_Abs_Long_Velocity>"
  Bus Selector/11 -> Subsystem1/2(<OBJ_Abs_Long_Velocity_STD>)  "<OBJ_Abs_Long_Velocity_STD>"
  Bus Selector/12 -> Subsystem1/3(<OBJ_Abs_Lat_Velocity>)  "<OBJ_Abs_Lat_Velocity>"
  Bus Selector/13 -> Subsystem1/4(<OBJ_Abs_Lat_Velocity_STD>)  "<OBJ_Abs_Lat_Velocity_STD>"
  Subsystem1/1(Out1) -> Bus Creator1/8  "Obj_Vel"
  Bus Selector/14 -> Subsystem2/1(<OBJ_Angle_Mid>)  "<OBJ_Angle_Mid>"
  Bus Selector/15 -> Subsystem2/2(<OBJ_Angle_Mid_STD>)  "<OBJ_Angle_Mid_STD>"
  Subsystem2/1(Out1) -> Bus Creator1/9  "Obj_Anage"
  Bus Selector/16 -> Bus Creator1/10  "<OBJ_Inv_TTC>"
  Bus Selector/17 -> Bus Creator1/11  "<OBJ_Inv_TTC_STD>"
  Bus Selector/18 -> Subsystem3/1(<OBJ_Abs_Long_Acc>)  "<OBJ_Abs_Long_Acc>"
  Bus Selector/19 -> Subsystem3/2(<OBJ_Abs_Long_Acc_STD>)  "<OBJ_Abs_Long_Acc_STD>"
  Bus Selector/20 -> Subsystem3/3(<OBJ_Abs_Lat_Acc>)  "<OBJ_Abs_Lat_Acc>"
  Bus Selector/21 -> Subsystem3/4(<OBJ_Abs_Lat_Acc_STD>)  "<OBJ_Abs_Lat_Acc_STD>"
  Subsystem3/1(Out1) -> Bus Creator1/12  "Obj_Acc"
  Constant/1 -> Bus Creator1/13  "existProb"
  Bus Selector/22 -> Subsystem4/1(<OBJ_Length>)  "<OBJ_Length>"
  Bus Selector/23 -> Subsystem4/2(<OBJ_Width>)  "<OBJ_Width>"
  Bus Selector/24 -> Subsystem4/3(<OBJ_Height>)  "<OBJ_Height>"
  Subsystem4/1(Out1) -> Bus Creator1/14  "Obj_BoxSize"
  Constant1/1 -> Bus Creator1/15  "AngelOfObj"
  Subsystem5/1(reserved1) -> Bus Creator1/16
  Bus Selector/25 -> Bus Creator1/17  "<OBJ_Heading>"
  Constant2/1 -> Bus Creator1/18
  Constant3/1 -> Bus Creator1/19
  Constant4/1 -> Bus Creator1/20
  Subsystem6/1(reserved2) -> Bus Creator1/21
  EyeQ4_Obj_01/1 -> Bus Selector/1
  Bus Creator1/1 -> Obj_01_st/1
  Data Type Conversion/1 -> Bus Creator1/1
  Data Type Conversion3/1 -> Bus Creator1/6  "Obj_TypeConf"
  Bus Selector/2 -> Subsystem7/1(<OBJ_Measuring_Status>)  "<OBJ_Measuring_Status>"
  Subsystem7/1(Obj_Status) -> Bus Creator1/2  "Obj_Status"
  Bus Selector/4 -> Subsystem8/1(<OBJ_Object_Class>)  "<OBJ_Object_Class>"
  Subsystem8/1(Obj_Type) -> Bus Creator1/5  "Obj_Type"

== system fusionAlg/FUSION /FUS_DataAdapter/VisionAdapter/ObjAdapter/Obj_16 ==
  EyeQ4_Obj_01 : Inport
  Bus Creator1 : BusCreator  Inputs=21  OutDataTypeStr=Bus: FUS_VISION_OBJ_ST
      settings: InheritFromInputs=off
  Bus Selector : BusSelector  OutputSignals=OBJ_ID,OBJ_Measuring_Status,OBJ_Object_Age,OBJ_Object_Class,OBJ_Class_Probability,OBJ_Lat_Distance,OBJ_Lat_Distance_STD,OBJ_Long_Distance,OBJ_Long_Distance_STD,OBJ_Abs_Long_Velocity,OBJ_Abs_Long_Velocity_STD,OBJ_Abs_Lat_Velocity,OBJ_Abs_Lat_Velocity_STD,OBJ_Angle_Mid,OBJ_Angle_Mid_STD,OBJ_Inv_TTC,OBJ_Inv_TTC_STD,OBJ_Abs_Long_Acc,OBJ_Abs_Long_Acc_STD,OBJ_Abs_Lat_Acc,OBJ_Abs_Lat_Acc_STD,OBJ_Length,OBJ_Width,OBJ_Height,OBJ_Heading
  Constant : Constant  OutDataTypeStr=single
  Constant1 : Constant  Value=0  OutDataTypeStr=uint8
  Constant2 : Constant  OutDataTypeStr=single
  Constant3 : Constant  Value=0  OutDataTypeStr=single
  Constant4 : Constant  Value=0  OutDataTypeStr=single
  Data Type Conversion : DataTypeConversion  OutDataTypeStr=uint32
  Data Type Conversion3 : DataTypeConversion  OutDataTypeStr=uint32
  Obj_01_Agge : Subsystem
  Obj_01_boundarhy : Subsystem
  Subsystem : Subsystem
  Subsystem1 : Subsystem
  Subsystem2 : Subsystem
  Subsystem3 : Subsystem
  Subsystem4 : Subsystem
  Subsystem5 : Subsystem
  Subsystem6 : Subsystem
  Subsystem7 : Subsystem
  Subsystem8 : Subsystem
  Obj_01_st : Outport  OutDataTypeStr=Bus: FUS_VISION_OBJ_ST
  wires:
  Bus Selector/1 -> Data Type Conversion/1  "<OBJ_ID>"
  Bus Selector/3 -> Obj_01_Agge/1(<OBJ_Object_Age>)  "<OBJ_Object_Age>"
  Obj_01_Agge/1(Obj_01_Age) -> Bus Creator1/3  "Obj_Age"
  Obj_01_boundarhy/1(Obj_01_boundary) -> Bus Creator1/4  "Obj_Boundary"
  Bus Selector/5 -> Data Type Conversion3/1  "<OBJ_Class_Probability>"
  Bus Selector/6 -> Subsystem/1(<OBJ_Lat_Distance>)  "<OBJ_Lat_Distance>"
  Bus Selector/7 -> Subsystem/2(<OBJ_Lat_Distance_STD>)  "<OBJ_Lat_Distance_STD>"
  Bus Selector/8 -> Subsystem/3(<OBJ_Long_Distance>)  "<OBJ_Long_Distance>"
  Bus Selector/9 -> Subsystem/4(<OBJ_Long_Distance_STD>)  "<OBJ_Long_Distance_STD>"
  Subsystem/1(Obj_01_coordinate) -> Bus Creator1/7  "Obj_Coor"
  Bus Selector/10 -> Subsystem1/1(<OBJ_Abs_Long_Velocity>)  "<OBJ_Abs_Long_Velocity>"
  Bus Selector/11 -> Subsystem1/2(<OBJ_Abs_Long_Velocity_STD>)  "<OBJ_Abs_Long_Velocity_STD>"
  Bus Selector/12 -> Subsystem1/3(<OBJ_Abs_Lat_Velocity>)  "<OBJ_Abs_Lat_Velocity>"
  Bus Selector/13 -> Subsystem1/4(<OBJ_Abs_Lat_Velocity_STD>)  "<OBJ_Abs_Lat_Velocity_STD>"
  Subsystem1/1(Out1) -> Bus Creator1/8  "Obj_Vel"
  Bus Selector/14 -> Subsystem2/1(<OBJ_Angle_Mid>)  "<OBJ_Angle_Mid>"
  Bus Selector/15 -> Subsystem2/2(<OBJ_Angle_Mid_STD>)  "<OBJ_Angle_Mid_STD>"
  Subsystem2/1(Out1) -> Bus Creator1/9  "Obj_Anage"
  Bus Selector/16 -> Bus Creator1/10  "<OBJ_Inv_TTC>"
  Bus Selector/17 -> Bus Creator1/11  "<OBJ_Inv_TTC_STD>"
  Bus Selector/18 -> Subsystem3/1(<OBJ_Abs_Long_Acc>)  "<OBJ_Abs_Long_Acc>"
  Bus Selector/19 -> Subsystem3/2(<OBJ_Abs_Long_Acc_STD>)  "<OBJ_Abs_Long_Acc_STD>"
  Bus Selector/20 -> Subsystem3/3(<OBJ_Abs_Lat_Acc>)  "<OBJ_Abs_Lat_Acc>"
  Bus Selector/21 -> Subsystem3/4(<OBJ_Abs_Lat_Acc_STD>)  "<OBJ_Abs_Lat_Acc_STD>"
  Subsystem3/1(Out1) -> Bus Creator1/12  "Obj_Acc"
  Constant/1 -> Bus Creator1/13  "existProb"
  Bus Selector/22 -> Subsystem4/1(<OBJ_Length>)  "<OBJ_Length>"
  Bus Selector/23 -> Subsystem4/2(<OBJ_Width>)  "<OBJ_Width>"
  Bus Selector/24 -> Subsystem4/3(<OBJ_Height>)  "<OBJ_Height>"
  Subsystem4/1(Out1) -> Bus Creator1/14  "Obj_BoxSize"
  Constant1/1 -> Bus Creator1/15  "AngelOfObj"
  Subsystem5/1(reserved1) -> Bus Creator1/16
  Bus Selector/25 -> Bus Creator1/17  "<OBJ_Heading>"
  Constant2/1 -> Bus Creator1/18
  Constant3/1 -> Bus Creator1/19
  Constant4/1 -> Bus Creator1/20
  Subsystem6/1(reserved2) -> Bus Creator1/21
  EyeQ4_Obj_01/1 -> Bus Selector/1
  Bus Creator1/1 -> Obj_01_st/1
  Data Type Conversion/1 -> Bus Creator1/1
  Data Type Conversion3/1 -> Bus Creator1/6  "Obj_TypeConf"
  Bus Selector/2 -> Subsystem7/1(<OBJ_Measuring_Status>)  "<OBJ_Measuring_Status>"
  Subsystem7/1(Obj_Status) -> Bus Creator1/2  "Obj_Status"
  Bus Selector/4 -> Subsystem8/1(<OBJ_Object_Class>)  "<OBJ_Object_Class>"
  Subsystem8/1(Obj_Type) -> Bus Creator1/5  "Obj_Type"

== system fusionAlg/FUSION /FUS_DataAdapter/VisionAdapter/ObjAdapter/Obj_17 ==
  EyeQ4_Obj_01 : Inport
  Bus Creator1 : BusCreator  Inputs=21  OutDataTypeStr=Bus: FUS_VISION_OBJ_ST
      settings: InheritFromInputs=off
  Bus Selector : BusSelector  OutputSignals=OBJ_ID,OBJ_Measuring_Status,OBJ_Object_Age,OBJ_Object_Class,OBJ_Class_Probability,OBJ_Lat_Distance,OBJ_Lat_Distance_STD,OBJ_Long_Distance,OBJ_Long_Distance_STD,OBJ_Abs_Long_Velocity,OBJ_Abs_Long_Velocity_STD,OBJ_Abs_Lat_Velocity,OBJ_Abs_Lat_Velocity_STD,OBJ_Angle_Mid,OBJ_Angle_Mid_STD,OBJ_Inv_TTC,OBJ_Inv_TTC_STD,OBJ_Abs_Long_Acc,OBJ_Abs_Long_Acc_STD,OBJ_Abs_Lat_Acc,OBJ_Abs_Lat_Acc_STD,OBJ_Length,OBJ_Width,OBJ_Height,OBJ_Heading
  Constant : Constant  OutDataTypeStr=single
  Constant1 : Constant  Value=0  OutDataTypeStr=uint8
  Constant2 : Constant  OutDataTypeStr=single
  Constant3 : Constant  Value=0  OutDataTypeStr=single
  Constant4 : Constant  Value=0  OutDataTypeStr=single
  Data Type Conversion : DataTypeConversion  OutDataTypeStr=uint32
  Data Type Conversion3 : DataTypeConversion  OutDataTypeStr=uint32
  Obj_01_Agge : Subsystem
  Obj_01_boundarhy : Subsystem
  Subsystem : Subsystem
  Subsystem1 : Subsystem
  Subsystem2 : Subsystem
  Subsystem3 : Subsystem
  Subsystem4 : Subsystem
  Subsystem5 : Subsystem
  Subsystem6 : Subsystem
  Subsystem7 : Subsystem
  Subsystem8 : Subsystem
  Obj_01_st : Outport  OutDataTypeStr=Bus: FUS_VISION_OBJ_ST
  wires:
  Bus Selector/1 -> Data Type Conversion/1  "<OBJ_ID>"
  Bus Selector/3 -> Obj_01_Agge/1(<OBJ_Object_Age>)  "<OBJ_Object_Age>"
  Obj_01_Agge/1(Obj_01_Age) -> Bus Creator1/3  "Obj_Age"
  Obj_01_boundarhy/1(Obj_01_boundary) -> Bus Creator1/4  "Obj_Boundary"
  Bus Selector/5 -> Data Type Conversion3/1  "<OBJ_Class_Probability>"
  Bus Selector/6 -> Subsystem/1(<OBJ_Lat_Distance>)  "<OBJ_Lat_Distance>"
  Bus Selector/7 -> Subsystem/2(<OBJ_Lat_Distance_STD>)  "<OBJ_Lat_Distance_STD>"
  Bus Selector/8 -> Subsystem/3(<OBJ_Long_Distance>)  "<OBJ_Long_Distance>"
  Bus Selector/9 -> Subsystem/4(<OBJ_Long_Distance_STD>)  "<OBJ_Long_Distance_STD>"
  Subsystem/1(Obj_01_coordinate) -> Bus Creator1/7  "Obj_Coor"
  Bus Selector/10 -> Subsystem1/1(<OBJ_Abs_Long_Velocity>)  "<OBJ_Abs_Long_Velocity>"
  Bus Selector/11 -> Subsystem1/2(<OBJ_Abs_Long_Velocity_STD>)  "<OBJ_Abs_Long_Velocity_STD>"
  Bus Selector/12 -> Subsystem1/3(<OBJ_Abs_Lat_Velocity>)  "<OBJ_Abs_Lat_Velocity>"
  Bus Selector/13 -> Subsystem1/4(<OBJ_Abs_Lat_Velocity_STD>)  "<OBJ_Abs_Lat_Velocity_STD>"
  Subsystem1/1(Out1) -> Bus Creator1/8  "Obj_Vel"
  Bus Selector/14 -> Subsystem2/1(<OBJ_Angle_Mid>)  "<OBJ_Angle_Mid>"
  Bus Selector/15 -> Subsystem2/2(<OBJ_Angle_Mid_STD>)  "<OBJ_Angle_Mid_STD>"
  Subsystem2/1(Out1) -> Bus Creator1/9  "Obj_Anage"
  Bus Selector/16 -> Bus Creator1/10  "<OBJ_Inv_TTC>"
  Bus Selector/17 -> Bus Creator1/11  "<OBJ_Inv_TTC_STD>"
  Bus Selector/18 -> Subsystem3/1(<OBJ_Abs_Long_Acc>)  "<OBJ_Abs_Long_Acc>"
  Bus Selector/19 -> Subsystem3/2(<OBJ_Abs_Long_Acc_STD>)  "<OBJ_Abs_Long_Acc_STD>"
  Bus Selector/20 -> Subsystem3/3(<OBJ_Abs_Lat_Acc>)  "<OBJ_Abs_Lat_Acc>"
  Bus Selector/21 -> Subsystem3/4(<OBJ_Abs_Lat_Acc_STD>)  "<OBJ_Abs_Lat_Acc_STD>"
  Subsystem3/1(Out1) -> Bus Creator1/12  "Obj_Acc"
  Constant/1 -> Bus Creator1/13  "existProb"
  Bus Selector/22 -> Subsystem4/1(<OBJ_Length>)  "<OBJ_Length>"
  Bus Selector/23 -> Subsystem4/2(<OBJ_Width>)  "<OBJ_Width>"
  Bus Selector/24 -> Subsystem4/3(<OBJ_Height>)  "<OBJ_Height>"
  Subsystem4/1(Out1) -> Bus Creator1/14  "Obj_BoxSize"
  Constant1/1 -> Bus Creator1/15  "AngelOfObj"
  Subsystem5/1(reserved1) -> Bus Creator1/16
  Bus Selector/25 -> Bus Creator1/17  "<OBJ_Heading>"
  Constant2/1 -> Bus Creator1/18
  Constant3/1 -> Bus Creator1/19
  Constant4/1 -> Bus Creator1/20
  Subsystem6/1(reserved2) -> Bus Creator1/21
  EyeQ4_Obj_01/1 -> Bus Selector/1
  Bus Creator1/1 -> Obj_01_st/1
  Data Type Conversion/1 -> Bus Creator1/1
  Data Type Conversion3/1 -> Bus Creator1/6  "Obj_TypeConf"
  Bus Selector/2 -> Subsystem7/1(<OBJ_Measuring_Status>)  "<OBJ_Measuring_Status>"
  Subsystem7/1(Obj_Status) -> Bus Creator1/2  "Obj_Status"
  Bus Selector/4 -> Subsystem8/1(<OBJ_Object_Class>)  "<OBJ_Object_Class>"
  Subsystem8/1(Obj_Type) -> Bus Creator1/5  "Obj_Type"

== system fusionAlg/FUSION /FUS_DataAdapter/VisionAdapter/ObjAdapter/Obj_18 ==
  EyeQ4_Obj_01 : Inport
  Bus Creator1 : BusCreator  Inputs=21  OutDataTypeStr=Bus: FUS_VISION_OBJ_ST
      settings: InheritFromInputs=off
  Bus Selector : BusSelector  OutputSignals=OBJ_ID,OBJ_Measuring_Status,OBJ_Object_Age,OBJ_Object_Class,OBJ_Class_Probability,OBJ_Lat_Distance,OBJ_Lat_Distance_STD,OBJ_Long_Distance,OBJ_Long_Distance_STD,OBJ_Abs_Long_Velocity,OBJ_Abs_Long_Velocity_STD,OBJ_Abs_Lat_Velocity,OBJ_Abs_Lat_Velocity_STD,OBJ_Angle_Mid,OBJ_Angle_Mid_STD,OBJ_Inv_TTC,OBJ_Inv_TTC_STD,OBJ_Abs_Long_Acc,OBJ_Abs_Long_Acc_STD,OBJ_Abs_Lat_Acc,OBJ_Abs_Lat_Acc_STD,OBJ_Length,OBJ_Width,OBJ_Height,OBJ_Heading
  Constant : Constant  OutDataTypeStr=single
  Constant1 : Constant  Value=0  OutDataTypeStr=uint8
  Constant2 : Constant  OutDataTypeStr=single
  Constant3 : Constant  Value=0  OutDataTypeStr=single
  Constant4 : Constant  Value=0  OutDataTypeStr=single
  Data Type Conversion : DataTypeConversion  OutDataTypeStr=uint32
  Data Type Conversion3 : DataTypeConversion  OutDataTypeStr=uint32
  Obj_01_Agge : Subsystem
  Obj_01_boundarhy : Subsystem
  Subsystem : Subsystem
  Subsystem1 : Subsystem
  Subsystem2 : Subsystem
  Subsystem3 : Subsystem
  Subsystem4 : Subsystem
  Subsystem5 : Subsystem
  Subsystem6 : Subsystem
  Subsystem7 : Subsystem
  Subsystem8 : Subsystem
  Obj_01_st : Outport  OutDataTypeStr=Bus: FUS_VISION_OBJ_ST
  wires:
  Bus Selector/1 -> Data Type Conversion/1  "<OBJ_ID>"
  Bus Selector/3 -> Obj_01_Agge/1(<OBJ_Object_Age>)  "<OBJ_Object_Age>"
  Obj_01_Agge/1(Obj_01_Age) -> Bus Creator1/3  "Obj_Age"
  Obj_01_boundarhy/1(Obj_01_boundary) -> Bus Creator1/4  "Obj_Boundary"
  Bus Selector/5 -> Data Type Conversion3/1  "<OBJ_Class_Probability>"
  Bus Selector/6 -> Subsystem/1(<OBJ_Lat_Distance>)  "<OBJ_Lat_Distance>"
  Bus Selector/7 -> Subsystem/2(<OBJ_Lat_Distance_STD>)  "<OBJ_Lat_Distance_STD>"
  Bus Selector/8 -> Subsystem/3(<OBJ_Long_Distance>)  "<OBJ_Long_Distance>"
  Bus Selector/9 -> Subsystem/4(<OBJ_Long_Distance_STD>)  "<OBJ_Long_Distance_STD>"
  Subsystem/1(Obj_01_coordinate) -> Bus Creator1/7  "Obj_Coor"
  Bus Selector/10 -> Subsystem1/1(<OBJ_Abs_Long_Velocity>)  "<OBJ_Abs_Long_Velocity>"
  Bus Selector/11 -> Subsystem1/2(<OBJ_Abs_Long_Velocity_STD>)  "<OBJ_Abs_Long_Velocity_STD>"
  Bus Selector/12 -> Subsystem1/3(<OBJ_Abs_Lat_Velocity>)  "<OBJ_Abs_Lat_Velocity>"
  Bus Selector/13 -> Subsystem1/4(<OBJ_Abs_Lat_Velocity_STD>)  "<OBJ_Abs_Lat_Velocity_STD>"
  Subsystem1/1(Out1) -> Bus Creator1/8  "Obj_Vel"
  Bus Selector/14 -> Subsystem2/1(<OBJ_Angle_Mid>)  "<OBJ_Angle_Mid>"
  Bus Selector/15 -> Subsystem2/2(<OBJ_Angle_Mid_STD>)  "<OBJ_Angle_Mid_STD>"
  Subsystem2/1(Out1) -> Bus Creator1/9  "Obj_Anage"
  Bus Selector/16 -> Bus Creator1/10  "<OBJ_Inv_TTC>"
  Bus Selector/17 -> Bus Creator1/11  "<OBJ_Inv_TTC_STD>"
  Bus Selector/18 -> Subsystem3/1(<OBJ_Abs_Long_Acc>)  "<OBJ_Abs_Long_Acc>"
  Bus Selector/19 -> Subsystem3/2(<OBJ_Abs_Long_Acc_STD>)  "<OBJ_Abs_Long_Acc_STD>"
  Bus Selector/20 -> Subsystem3/3(<OBJ_Abs_Lat_Acc>)  "<OBJ_Abs_Lat_Acc>"
  Bus Selector/21 -> Subsystem3/4(<OBJ_Abs_Lat_Acc_STD>)  "<OBJ_Abs_Lat_Acc_STD>"
  Subsystem3/1(Out1) -> Bus Creator1/12  "Obj_Acc"
  Constant/1 -> Bus Creator1/13  "existProb"
  Bus Selector/22 -> Subsystem4/1(<OBJ_Length>)  "<OBJ_Length>"
  Bus Selector/23 -> Subsystem4/2(<OBJ_Width>)  "<OBJ_Width>"
  Bus Selector/24 -> Subsystem4/3(<OBJ_Height>)  "<OBJ_Height>"
  Subsystem4/1(Out1) -> Bus Creator1/14  "Obj_BoxSize"
  Constant1/1 -> Bus Creator1/15  "AngelOfObj"
  Subsystem5/1(reserved1) -> Bus Creator1/16
  Bus Selector/25 -> Bus Creator1/17  "<OBJ_Heading>"
  Constant2/1 -> Bus Creator1/18
  Constant3/1 -> Bus Creator1/19
  Constant4/1 -> Bus Creator1/20
  Subsystem6/1(reserved2) -> Bus Creator1/21
  EyeQ4_Obj_01/1 -> Bus Selector/1
  Bus Creator1/1 -> Obj_01_st/1
  Data Type Conversion/1 -> Bus Creator1/1
  Data Type Conversion3/1 -> Bus Creator1/6  "Obj_TypeConf"
  Bus Selector/2 -> Subsystem7/1(<OBJ_Measuring_Status>)  "<OBJ_Measuring_Status>"
  Subsystem7/1(Obj_Status) -> Bus Creator1/2  "Obj_Status"
  Bus Selector/4 -> Subsystem8/1(<OBJ_Object_Class>)  "<OBJ_Object_Class>"
  Subsystem8/1(Obj_Type) -> Bus Creator1/5  "Obj_Type"
